simulink model "FM_audio_Tx_Rx_baseband"  (R2026a)
settings: Solver=VariableStepAuto  StopTime=inf
model workspace (MAT data in the model file):
  Kf = 20000
libraries: commanabbnd3 x2, commchan3 x1, dspsnks4 x1, dspvision x1, dspfdesign x1, commrflib2 x1
settings Model: Creator=ranja  LastModifiedBy=ranja

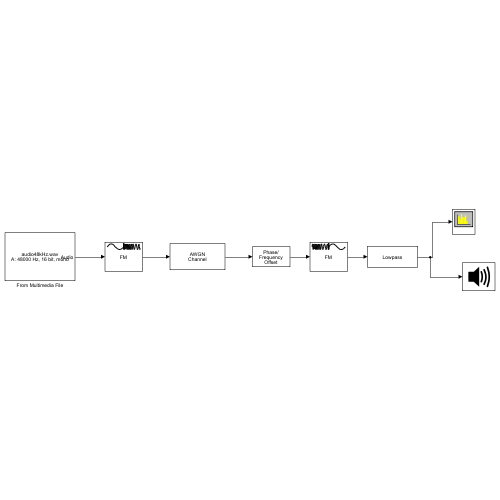
[thumbnail: Simulink's stored preview of the top-level diagram]
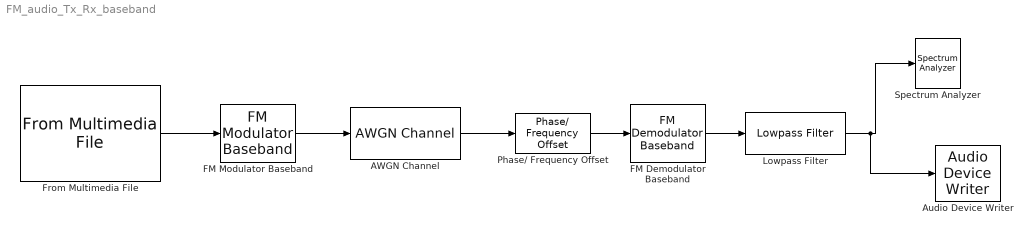
== system FM_audio_Tx_Rx_baseband ==
  AWGN Channel : commchan3/AWGN Channel  LegacyMode=off  NoiseMethod="Signal to noise ratio  (SNR)"  noiseMode="Signal to noise ratio  (SNR)"  EbNo=10  EsNo=10  SNR=30  BitsPerSymbol=1  SignalPower=1  SpecifySymbolPeriod=off  SamplesPerSymbol=1  SymbolPeriod=1  VarianceSource=Parameter  Variance=1  RandomStream=Global stream  Seed=67  SimulateUsing=Code generation
  Audio Device Writer : dspsnks4/Audio Device Writer  Driver=DirectSound  Device=Default  InheritSampleRate=on  SampleRate=44100  BitDepth=16-bit integer  BufferSize=4096  NumBuffers=10  DefaultOutputChannelMapping=on  OutputChannelMapping=1:2  OutputNumUnderrunSamples=off  DriverIdx=1  DeviceWarnFlag=''
  "FM Demodulator Baseband " : commanabbnd3/FM Demodulator Baseband   FrequencyDeviation=Kf  SimulateUsing=Code generation
  FM Modulator Baseband : commanabbnd3/FM Modulator Baseband  FrequencyDeviation=20e3  SimulateUsing=Code generation
  From Multimedia File : dspvision/From Multimedia File  inputFilename=C:\Program Files\MATLAB\R2026a\toolbox\dsp\dsp\samples\audio48kHz.wav  readRange=[1 Inf]  loop=on  numPlays=inf  outputStreams=Audio only  videoDataType=single  audioDataType=double  inheritSampleTime=on  userDefinedSampleTime=1/30  noAudioOutput=off  isIntensityVideo=off  fourcc=RGB  colorVideoFormat=One multidimensional signal  outputEOF=off  dataOrg=Column-major  audioFrameSize=1024  computeAudioFrameSize=off  outSamplingMode=Sample based
      settings: LibrarySourceBlock=dspsrcs4/From Multimedia File
  Lowpass Filter : dspfdesign/Lowpass Filter  FilterType=FIR  DesignForMinimumOrder=off  FilterOrder=50  PassbandFrequency=6000  StopbandFrequency=0.5442  PassbandRipple=0.1  StopbandAttenuation=80  SampleRateMode=Specify on dialog  SampleRate=48000  SimulateUsing=Interpreted execution  roundingMode=Floor  coeffsDataTypeStr=fixdt(1,16)
  Phase/ Frequency Offset : commrflib2/Phase// Frequency Offset  PhaseOffset=0  FrequencyOffsetFromPort=off  FrequencyOffset=0  SimulateUsing=Code generation
  Spectrum Analyzer : SpectrumAnalyzer  WindowInvariantSamplesPerUpdate=on
  wires:
  From Multimedia File/1 -> FM Modulator Baseband/1
  FM Modulator Baseband/1 -> AWGN Channel/1
  AWGN Channel/1 -> Phase/ Frequency Offset/1
  Phase/ Frequency Offset/1 -> "FM Demodulator Baseband "/1
  "FM Demodulator Baseband "/1 -> Lowpass Filter/1
  Lowpass Filter/1 -> Audio Device Writer/1, Spectrum Analyzer/1
